simulink model "EurlerDynJointVerifyIdn"  (Simulink 7.6)
settings: Solver=ode45  StartTime=0.0  StopTime=8  RelTol=1e-3
InitFcn:
  | eval('Config')
values from neighbouring files (symbols this model uses):
  a2 = 0    [Config.m]    (also in CtrPlatformCfg.m)
  a3 = 0    [Config.m]    (also in CtrPlatformCfg.m)
  a4 = 0    [Config.m]    (also in CtrPlatformCfg.m)
  a5 = 90    [Config.m]    (also in CtrPlatformCfg.m)
  a6 = 0    [Config.m]    (also in CtrPlatformCfg.m)
  DH_EU = [266     300     0       0       1016     0      174 ... (first row only)    [DynEulerTest.m]
  freq = tvel/radius    (= 1)    [Config.m]    (also in CtrPlatformCfg.m)
  Ft_EU = [0;0;0;0;0;0]    [DynEulerTest.m]
  init_Endx = gd_init(1,4)    [Config.m]    (also in CtrPlatformCfg.m)
  init_Endy = gd_init(2,4)    [Config.m]    (also in CtrPlatformCfg.m)
  init_Endz = gd_init(3,4)    [Config.m]    (also in CtrPlatformCfg.m)
  init_Rot = gd_init(1:3,1:3)    [Config.m]    (also in CtrPlatformCfg.m)
  L = [l1 l2 l3 l4 l5 l6 l7 l8 l9]    [Config.m]    (also in CtrPlatformCfg.m)
  tvel = 120    [Config.m]    (also in CtrPlatformCfg.m)
undefined symbols (not defined in the file or in its folder): a1, DH_Min, Ft_Min, Param_EU, Param_Min
libraries: mblibv1 x35, simulink x9
(part 1 of 2)
settings Model: Creator=DAI Dan  LastModifiedBy=DAI Dan
settings SimMechanicsCC: VisOnUpdateDiagram=on  VisDuringSimulation=on

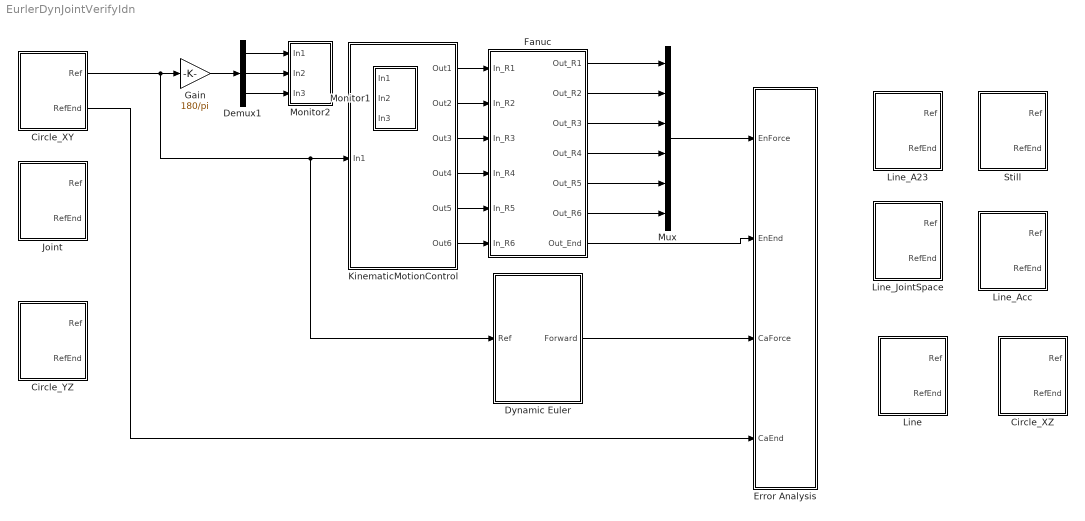
== system EurlerDynJointVerifyIdn ==
  Circle_XY : Subsystem
  Circle_XZ : Subsystem
  Circle_YZ : Subsystem
  Demux1 : Demux  Outputs=3
  Dynamic Euler : Subsystem
  Error Analysis : Subsystem
  Fanuc : Subsystem
  Gain : Gain  Gain=180/pi
  Joint : Subsystem
  KinematicMotionControl : Subsystem
  Line : Subsystem
  Line_A23 : Subsystem
  Line_Acc : Subsystem
  Line_JointSpace : Subsystem
  Monitor1 : Subsystem
  Monitor2 : Subsystem
  Mux : Mux  Inputs=6
  Still : Subsystem
  wires:
  KinematicMotionControl/1(Out1) -> Fanuc/1(In_R1)
  KinematicMotionControl/2(Out2) -> Fanuc/2(In_R2)
  KinematicMotionControl/3(Out3) -> Fanuc/3(In_R3)
  KinematicMotionControl/4(Out4) -> Fanuc/4(In_R4)
  KinematicMotionControl/5(Out5) -> Fanuc/5(In_R5)
  KinematicMotionControl/6(Out6) -> Fanuc/6(In_R6)
  Fanuc/5(Out_R5) -> Mux/5
  Fanuc/6(Out_R6) -> Mux/6
  Mux/1 -> Error Analysis/1(EnForce)
  Fanuc/4(Out_R4) -> Mux/4
  Fanuc/3(Out_R3) -> Mux/3
  Fanuc/2(Out_R2) -> Mux/2
  Fanuc/1(Out_R1) -> Mux/1
  Fanuc/7(Out_End) -> Error Analysis/2(EnEnd)
  Dynamic Euler/1(Forward) -> Error Analysis/3(CaForce)
  Demux1/1 -> Monitor2/1(In1)
  Demux1/2 -> Monitor2/2(In2)
  Demux1/3 -> Monitor2/3(In3)
  Gain/1 -> Demux1/1
  Circle_XY/1(Ref) -> Gain/1, KinematicMotionControl/1(In1), Dynamic Euler/1(Ref)
  Circle_XY/2(RefEnd) -> Error Analysis/4(CaEnd)

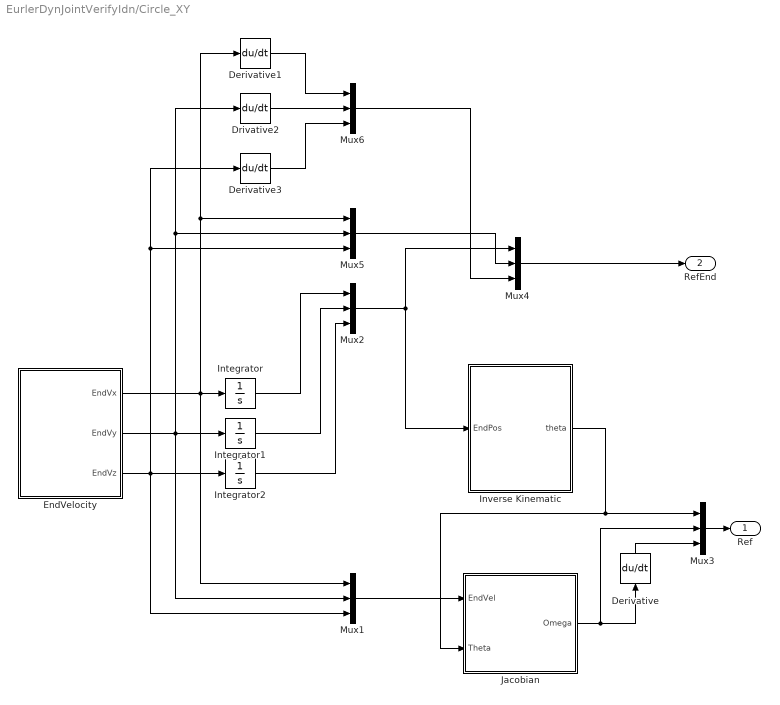
== system EurlerDynJointVerifyIdn/Circle_XY ==
  Derivative : Derivative
  Derivative1 : Derivative
  Derivative3 : Derivative
  Drivative2 : Derivative
  EndVelocity : Subsystem
  Integrator : Integrator  InitialCondition=init_Endx
  Integrator1 : Integrator  InitialCondition=init_Endy
  Integrator2 : Integrator  InitialCondition=init_Endz
  Inverse Kinematic : Stateflow chart  TreatAsAtomicUnit=on
  Jacobian : Stateflow chart  TreatAsAtomicUnit=on
  Mux{1..6} (6 alike) : Mux  Inputs=3
  Ref : Outport
  RefEnd : Outport  Port=2
  wires:
  Integrator/1 -> Mux2/1
  Integrator1/1 -> Mux2/2
  EndVelocity/1(EndVx) -> Integrator/1, Mux1/1, Mux5/1, Derivative1/1
  EndVelocity/2(EndVy) -> Integrator1/1, Mux1/2, Mux5/2, Drivative2/1
  EndVelocity/3(EndVz) -> Integrator2/1, Mux1/3, Mux5/3, Derivative3/1
  Integrator2/1 -> Mux2/3
  Mux2/1 -> Mux4/1, Inverse Kinematic/1(EndPos)
  Mux1/1 -> Jacobian/1(EndVel)
  Jacobian/1(Omega) -> Mux3/2, Derivative/1
  Mux3/1 -> Ref/1
  Derivative/1 -> Mux3/3
  Inverse Kinematic/1(theta) -> Mux3/1, Jacobian/2(Theta)
  Mux5/1 -> Mux4/2
  Mux4/1 -> RefEnd/1
  Derivative1/1 -> Mux6/1
  Drivative2/1 -> Mux6/2
  Derivative3/1 -> Mux6/3
  Mux6/1 -> Mux4/3

== system EurlerDynJointVerifyIdn/Circle_XZ ==
  Derivative : Derivative
  Derivative1 : Derivative
  Derivative3 : Derivative
  Drivative2 : Derivative
  EndVelocity : Subsystem
  Integrator : Integrator  InitialCondition=init_Endx
  Integrator1 : Integrator  InitialCondition=init_Endy
  Integrator2 : Integrator  InitialCondition=init_Endz
  Inverse Kinematic : Stateflow chart  TreatAsAtomicUnit=on
  Jacobian : Stateflow chart  TreatAsAtomicUnit=on
  Mux{1..6} (6 alike) : Mux  Inputs=3
  Ref : Outport
  RefEnd : Outport  Port=2
  wires:
  Integrator/1 -> Mux2/1
  Integrator1/1 -> Mux2/2
  EndVelocity/1(EndVx) -> Integrator/1, Mux1/1, Mux5/1, Derivative1/1
  EndVelocity/2(EndVy) -> Integrator1/1, Mux1/2, Mux5/2, Drivative2/1
  EndVelocity/3(EndVz) -> Integrator2/1, Mux1/3, Mux5/3, Derivative3/1
  Integrator2/1 -> Mux2/3
  Mux2/1 -> Mux4/1, Inverse Kinematic/1(EndPos)
  Mux1/1 -> Jacobian/1(EndVel)
  Jacobian/1(Omega) -> Mux3/2, Derivative/1
  Mux3/1 -> Ref/1
  Derivative/1 -> Mux3/3
  Inverse Kinematic/1(theta) -> Mux3/1, Jacobian/2(Theta)
  Mux5/1 -> Mux4/2
  Mux4/1 -> RefEnd/1
  Derivative1/1 -> Mux6/1
  Drivative2/1 -> Mux6/2
  Derivative3/1 -> Mux6/3
  Mux6/1 -> Mux4/3

== system EurlerDynJointVerifyIdn/Circle_YZ ==
  Derivative : Derivative
  Derivative1 : Derivative
  Derivative3 : Derivative
  Drivative2 : Derivative
  EndVelocity : Subsystem
  Integrator : Integrator  InitialCondition=init_Endx
  Integrator1 : Integrator  InitialCondition=init_Endy
  Integrator2 : Integrator  InitialCondition=init_Endz
  Inverse Kinematic : Stateflow chart  TreatAsAtomicUnit=on
  Jacobian : Stateflow chart  TreatAsAtomicUnit=on
  Mux{1..6} (6 alike) : Mux  Inputs=3
  Ref : Outport
  RefEnd : Outport  Port=2
  wires:
  Integrator/1 -> Mux2/1
  Integrator1/1 -> Mux2/2
  EndVelocity/1(EndVx) -> Integrator/1, Mux1/1, Mux5/1, Derivative1/1
  EndVelocity/2(EndVy) -> Integrator1/1, Mux1/2, Mux5/2, Drivative2/1
  EndVelocity/3(EndVz) -> Integrator2/1, Mux1/3, Mux5/3, Derivative3/1
  Integrator2/1 -> Mux2/3
  Mux2/1 -> Mux4/1, Inverse Kinematic/1(EndPos)
  Mux1/1 -> Jacobian/1(EndVel)
  Jacobian/1(Omega) -> Mux3/2, Derivative/1
  Mux3/1 -> Ref/1
  Derivative/1 -> Mux3/3
  Inverse Kinematic/1(theta) -> Mux3/1, Jacobian/2(Theta)
  Mux5/1 -> Mux4/2
  Mux4/1 -> RefEnd/1
  Derivative1/1 -> Mux6/1
  Drivative2/1 -> Mux6/2
  Derivative3/1 -> Mux6/3
  Mux6/1 -> Mux4/3

== system EurlerDynJointVerifyIdn/Dynamic Euler ==
  Ref : Inport
  Demux : Demux  Outputs=3
  Newton Euler Recursion : Stateflow chart  TreatAsAtomicUnit=on
  Newton Euler Recursion1 : Stateflow chart  TreatAsAtomicUnit=on
  To Workspace : ToWorkspace  VariableName=OutAngle1  SaveFormat=Structure With Time
  To Workspace1 : ToWorkspace  VariableName=OutOmega1  SaveFormat=Structure With Time
  To Workspace2 : ToWorkspace  VariableName=OutAcc1  SampleTime=-1  SaveFormat=Structure With Time
  Forward : Outport
  wires:
  Ref/1 -> Demux/1
  Demux/1 -> To Workspace/1, Newton Euler Recursion/1(Pos), Newton Euler Recursion1/1(Pos)
  Demux/2 -> To Workspace1/1, Newton Euler Recursion/2(Vel), Newton Euler Recursion1/2(Vel)
  Demux/3 -> To Workspace2/1, Newton Euler Recursion/3(Acc), Newton Euler Recursion1/3(Acc)
  Newton Euler Recursion1/1(Torque) -> Forward/1

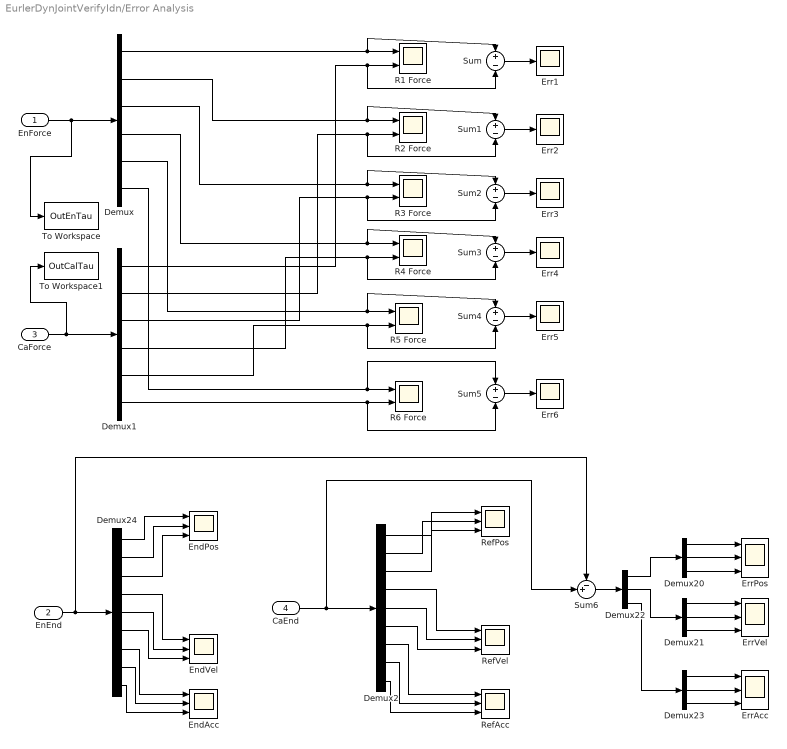
== system EurlerDynJointVerifyIdn/Error Analysis ==
  EnForce : Inport
  EnEnd : Inport  Port=2
  CaForce : Inport  Port=3
  CaEnd : Inport  Port=4
  Demux : Demux  Outputs=6
  Demux1 : Demux  Outputs=6
  Demux2 : Demux  Outputs=9
  Demux{20..23} (4 alike) : Demux  Outputs=3
  Demux24 : Demux  Outputs=9
  EndAcc : Scope  NumInputPorts=3
      settings: TimeRange=0.7279693486590038  YMin=-80~-80~0.03111111111111042  YMax=60~80~0.06666666666666621  SaveName=ScopeData12
  EndPos : Scope  NumInputPorts=3
      settings: TimeRange=10  YMin=1150~-100~1518.9999998  YMax=1350~200~1519.0000003  SaveName=ScopeData13
  EndVel : Scope  NumInputPorts=3
      settings: YMin=-5~-5~-5  YMax=5~5~5  SaveName=ScopeData14
  Err{1..6} (6 alike) : Scope
      Err1 settings: SaveName=ScopeData6
      Err2 settings: SaveName=ScopeData7
      Err3 settings: TimeRange=10  SaveName=ScopeData8
      Err4 settings: TimeRange=3  SaveName=ScopeData9
      Err5 settings: SaveName=ScopeData10
      Err6 settings: SaveName=ScopeData11
  ErrAcc : Scope  NumInputPorts=3
      settings: YMin=-5~-5~-5  YMax=5~5~5  SaveName=ScopeData15
  ErrPos : Scope  NumInputPorts=3
      settings: YMin=-5~-5~-5  YMax=5~5~5  SaveName=ScopeData16
  ErrVel : Scope  NumInputPorts=3
      settings: YMin=-5~-5~-5  YMax=5~5~5  SaveName=ScopeData17
  R1 Force : Scope  NumInputPorts=2
      settings: TimeRange=10  YMin=-2.999999999999999e-017~-1  YMax=4e-017~1
  R2 Force : Scope  NumInputPorts=2
      settings: YMin=-5~-5  YMax=5~5
  R3 Force : Scope  NumInputPorts=2
      settings: YMin=-5~-5  YMax=5~5  SaveName=ScopeData2
  R4 Force : Scope  NumInputPorts=2
      settings: TimeRange=8  YMin=-5~-5  YMax=5~5  SaveName=ScopeData3
  R5 Force : Scope  NumInputPorts=2
      settings: TimeRange=10  YMin=-4.18~4.060000000000001  YMax=-4.04~4.2  SaveName=ScopeData4
  R6 Force : Scope  NumInputPorts=2
      settings: TimeRange=10  YMin=-1.6e-006~-0.003  YMax=4e-007~0.004  SaveName=ScopeData5
  RefAcc : Scope  NumInputPorts=3
      settings: TimeRange=10  YMin=-5~-5~-5  YMax=5~5~5  SaveName=ScopeData18
  RefPos : Scope  NumInputPorts=3
      settings: YMin=-5~-5~-5  YMax=5~5~5  SaveName=ScopeData19
  RefVel : Scope  NumInputPorts=3
      settings: TimeRange=10  YMin=0~-1~-1  YMax=60~1~1  SaveName=ScopeData20
  Sum{,1..5} (6 alike) : Sum  Inputs=+|-
  Sum6 : Sum  Inputs=-+|
  To Workspace : ToWorkspace  VariableName=OutEnTau  SampleTime=-1  SaveFormat=Structure
  To Workspace1 : ToWorkspace  VariableName=OutCalTau  SampleTime=-1  SaveFormat=Structure
  wires:
  Sum/1 -> Err1/1
  Sum1/1 -> Err2/1
  Sum2/1 -> Err3/1
  Sum3/1 -> Err4/1
  Sum4/1 -> Err5/1
  Sum5/1 -> Err6/1
  EnForce/1 -> Demux/1, To Workspace/1
  CaForce/1 -> Demux1/1, To Workspace1/1
  Demux/1 -> Sum/1, R1 Force/1
  Demux1/1 -> Sum/2, R1 Force/2
  Demux/2 -> R2 Force/1, Sum1/1
  Demux/3 -> R3 Force/1, Sum2/1
  Demux/4 -> R4 Force/1, Sum3/1
  Demux/5 -> R5 Force/1, Sum4/1
  Demux/6 -> Sum5/1, R6 Force/1
  Demux1/2 -> R2 Force/2, Sum1/2
  Demux1/3 -> R3 Force/2, Sum2/2
  Demux1/4 -> R4 Force/2, Sum3/2
  Demux1/5 -> R5 Force/2, Sum4/2
  Demux1/6 -> Sum5/2, R6 Force/2
  EnEnd/1 -> Sum6/1, Demux24/1
  CaEnd/1 -> Sum6/2, Demux2/1
  Demux20/1 -> ErrPos/1
  Demux20/2 -> ErrPos/2
  Demux20/3 -> ErrPos/3
  Sum6/1 -> Demux22/1
  Demux22/1 -> Demux20/1
  Demux22/2 -> Demux21/1
  Demux21/1 -> ErrVel/1
  Demux21/2 -> ErrVel/2
  Demux21/3 -> ErrVel/3
  Demux2/1 -> RefPos/1
  Demux2/2 -> RefPos/2
  Demux2/3 -> RefPos/3
  Demux2/4 -> RefVel/1
  Demux2/5 -> RefVel/2
  Demux2/6 -> RefVel/3
  Demux2/7 -> RefAcc/1
  Demux2/8 -> RefAcc/2
  Demux2/9 -> RefAcc/3
  Demux23/1 -> ErrAcc/1
  Demux23/2 -> ErrAcc/2
  Demux23/3 -> ErrAcc/3
  Demux22/3 -> Demux23/1
  Demux24/1 -> EndPos/1
  Demux24/2 -> EndPos/2
  Demux24/3 -> EndPos/3
  Demux24/4 -> EndVel/1
  Demux24/5 -> EndVel/2
  Demux24/6 -> EndVel/3
  Demux24/7 -> EndAcc/1
  Demux24/8 -> EndAcc/2
  Demux24/9 -> EndAcc/3

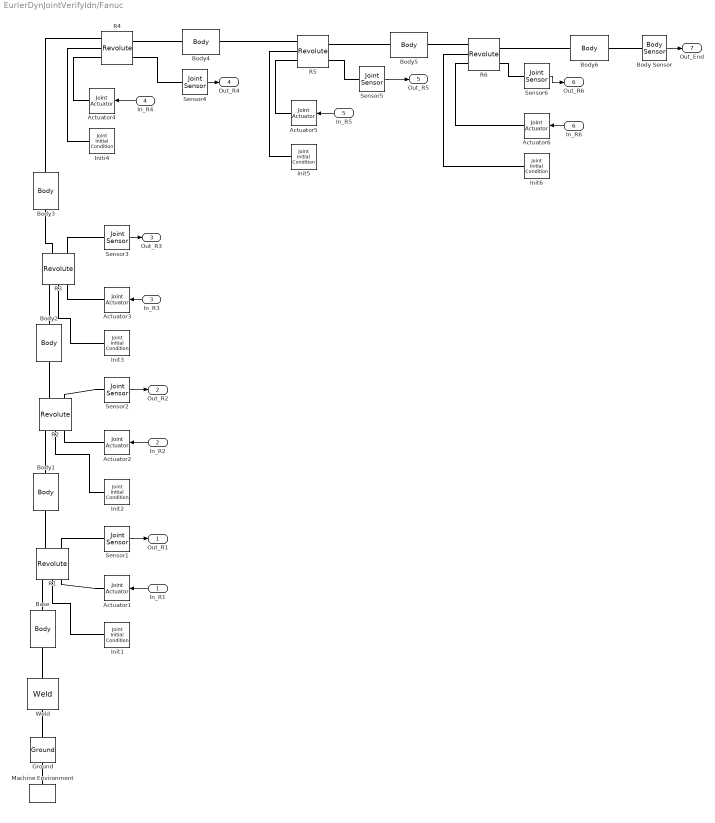
== system EurlerDynJointVerifyIdn/Fanuc ==
  In_R1 : Inport
  In_R2 : Inport  Port=2
  In_R3 : Inport  Port=3
  In_R4 : Inport  Port=4
  In_R5 : Inport  Port=5
  In_R6 : Inport  Port=6
  Actuator{1..6} (6 alike) : mblibv1/Sensors &  Actuators/Joint Actuator  DialogController=MECH.DynMechDlgSource  SystemSampleTime=-1  UpdateFromCAD=off  PhysicalDomain=Mechanical  PortType=blob  ActuationStyle=Motion  AngleUnits=rad  ArcVelocityUnits=rad/s  ArcAccelerationUnits=rad/s^2  CoordPositionUnits=m  VelocityUnits=m/s  AccelerationUnits=m/s^2  ForceUnits=N  TorqueUnits=N*m  ActiveIO=on  Width=3  DialogClass=MechanicalActuatorBlock  Primitive=R1  ReferenceFrame=Absolute (World)
  Base : mblibv1/Bodies/Body  DialogController=MECH.DynMechDlgSource  PhysicalDomain=mechanical  SubClassName=Unknown  LeftPortType=workingframe  RightPortType=workingframe  LConnTagsString=CS1  RConnTagsString=CS2  UpdateFromCAD=on  DialogClass=MechanicalBodyBlock  Mass=133.95  MassUnits=kg  InertiaUnits=kg*m^2  Inertia=[3.0977 0.0155 -0.0939;0.0155 3.3580 0.0061;-0.0939 0.0061 5.1969]  Shape=Cylinder  ShapeDims=[1 1]  ShapeUnits=m  ShapeUse=false  Density=1  DensityUnits=kg/m^3  DensityUse=false  GraphicsMode=GFXFILE  GraphicsFileName=M-710iC50 M-710iC70 - M-710iC50 M-710iC70 base-1.STL  BodyColorSelMode=COLORPALETTE  BodyColor=[0.25098 0.25098 0.25098]  AttachedToCS=CS1  CG=Right$CG$[-0.0437 -0.0026 0.1059]$WORLD$WORLD$m$[1 0 0;0 1 0;0 0 1]$3x3 Transform$rad$WORLD$false$none  WorkingFrames=Left$CS1$[0 0 0]$WORLD$WORLD$m$[1 0 0;0 1 0;0 0 1]$3x3 Transform$rad$WORLD$true$none#Right$CS2$[0 0 0.266]$WORLD$WORLD$m$[1 0 0;0 1 0;0 0 1]$3x3 Transform$rad$WORLD$true$none  CGPos=[-0.0437 -0.0026 0.1059]  CGRot=[1 0 0;0 1 0;0 0 1]  CS0Pos=[]  CS0Rot=[]  CS1Pos=[0 0 0]  CS1Rot=[1 0 0;0 1 0;0 0 1]  CS2Pos=[0 0 0.266]  CS2Rot=[1 0 0;0 1 0;0 0 1]  CS3Pos=[]  CS3Rot=[]  CS4Pos=[]  CS4Rot=[]  CS5Pos=[]  CS5Rot=[]  CS6Pos=[]  CS6Rot=[]  CS7Pos=[]  CS7Rot=[]  CS8Pos=[]  CS8Rot=[]  CS9Pos=[]  CS9Rot=[]  CS10Pos=[]  CS10Rot=[]  CS11Pos=[]  CS11Rot=[]  CS12Pos=[]  CS12Rot=[]  CS13Pos=[]  CS13Rot=[]  CS14Pos=[]  CS14Rot=[]  CS15Pos=[]  CS15Rot=[]  CS16Pos=[]  CS16Rot=[]  CS17Pos=[]  CS17Rot=[]  CS18Pos=[]  CS18Rot=[]  CS19Pos=[]  CS19Rot=[]  CS20Pos=[]  CS20Rot=[]
  Body Sensor : mblibv1/Sensors &  Actuators/Body Sensor  DialogController=MECH.DynMechDlgSource  SystemSampleTime=-1  UpdateFromCAD=off  PhysicalDomain=Mechanical  PortType=blob  Muxed=on  Pose=off  Angle=on  AngleUnits=deg  ArcVelocity=off  ArcVelocityUnits=deg/s  ArcAcceleration=off  ArcAccelerationUnits=deg/s^2  CoordPosition=on  CoordPositionUnits=mm  Velocity=on  VelocityUnits=mm/s  Acceleration=on  AccelerationUnits=mm/s^2  Quaternion=on  QuaternionDT=off  QuaternionDDT=off  QuaternionUnits=off  OutputVector=[1]  ActiveIO=on  Width=9  DialogClass=MechanicalSensorBlock  ReferenceFrame=Absolute (World)
  Body1 : mblibv1/Bodies/Body  DialogController=MECH.DynMechDlgSource  PhysicalDomain=mechanical  SubClassName=Unknown  LeftPortType=workingframe  RightPortType=workingframe  LConnTagsString=CS2  RConnTagsString=CS3  UpdateFromCAD=on  DialogClass=MechanicalBodyBlock  Mass=170.31  MassUnits=kg  InertiaUnits=kg*m^2  Inertia=[5.2954 -0.2565 -0.6366;-0.2565 4.7000 0.2830;-0.6366 0.2829 5.8635]  Shape=Cylinder  ShapeDims=[1 1]  ShapeUnits=m  ShapeUse=false  Density=1  DensityUnits=kg/m^3  DensityUse=false  GraphicsMode=GFXFILE  GraphicsFileName=M-710iC50 M-710iC70 - M-710iC50 M-710iC70 axis1-1.STL  BodyColorSelMode=COLORPALETTE  BodyColor=[0.86667 0.86667 0.8902]  AttachedToCS=CS1  CG=Right$CG$[0.0407 -0.0528 0.4702]$WORLD$WORLD$m$[1 0 0;0 1 0;0 0 1]$3x3 Transform$rad$WORLD$false$none  WorkingFrames=Right$CS1$[0 0 0]$WORLD$WORLD$m$[1 0 0;0 1 0;0 0 1]$3x3 Transform$rad$WORLD$false$none#Left$CS2$[0 0 0.266]$WORLD$WORLD$m$[1 0 0;0 1 0;0 0 1]$3x3 Transform$rad$WORLD$true$none#Right$CS3$[0.15 0.062 0.566]$WORLD$WORLD$m$[1 0 0;0 1 0;0 0 1]$3x3 Transform$rad$WORLD$true$none  CGPos=[0.0407 -0.0528 0.4702]  CGRot=[1 0 0;0 1 0;0 0 1]  CS0Pos=[]  CS0Rot=[]  CS1Pos=[0 0 0]  CS1Rot=[1 0 0;0 1 0;0 0 1]  CS2Pos=[0 0 0.266]  CS2Rot=[1 0 0;0 1 0;0 0 1]  CS3Pos=[0.15 0.062 0.566]  CS3Rot=[1 0 0;0 1 0;0 0 1]  CS4Pos=[]  CS4Rot=[]  CS5Pos=[]  CS5Rot=[]  CS6Pos=[]  CS6Rot=[]  CS7Pos=[]  CS7Rot=[]  CS8Pos=[]  CS8Rot=[]  CS9Pos=[]  CS9Rot=[]  CS10Pos=[]  CS10Rot=[]  CS11Pos=[]  CS11Rot=[]  CS12Pos=[]  CS12Rot=[]  CS13Pos=[]  CS13Rot=[]  CS14Pos=[]  CS14Rot=[]  CS15Pos=[]  CS15Rot=[]  CS16Pos=[]  CS16Rot=[]  CS17Pos=[]  CS17Rot=[]  CS18Pos=[]  CS18Rot=[]  CS19Pos=[]  CS19Rot=[]  CS20Pos=[]  CS20Rot=[]
  Body2 : mblibv1/Bodies/Body  DialogController=MECH.DynMechDlgSource  PhysicalDomain=mechanical  SubClassName=Unknown  LeftPortType=workingframe  RightPortType=workingframe  LConnTagsString=CS2  RConnTagsString=CS3  UpdateFromCAD=on  DialogClass=MechanicalBodyBlock  Mass=63.74  MassUnits=kg  InertiaUnits=kg*m^2  Inertia=[5.8840 0.0072 0.0135;0.0072 6.0178 -0.1907;0.0135 -0.1907 0.3374]  Shape=Cylinder  ShapeDims=[1 1]  ShapeUnits=m  ShapeUse=false  Density=1  DensityUnits=kg/m^3  DensityUse=false  GraphicsMode=GFXFILE  GraphicsFileName=M-710iC50 M-710iC70 - M-710iC50 M-710iC70 axis2-1.STL  BodyColorSelMode=COLORPALETTE  BodyColor=[1 1 0]  AttachedToCS=CS1  CG=Right$CG$[0.1510 0.1746 0.9687]$WORLD$WORLD$m$[1 0 0;0 1 0;0 0 1]$3x3 Transform$rad$WORLD$false$none  WorkingFrames=Right$CS1$[0 0 0]$WORLD$WORLD$m$[1 0 0;0 1 0;0 0 1]$3x3 Transform$rad$WORLD$false$none#Left$CS2$[0.15 0.062 0.566]$WORLD$WORLD$m$[1 0 0;0 1 0;0 0 1]$3x3 Transform$rad$WORLD$true$none#Right$CS3$[0.15 0.227 1.436]$WORLD$WORLD$m$[1 0 0;0 1 0;0 0 1]$3x3 Transform$rad$WORLD$true$none  CGPos=[0.1510 0.1746 0.9687]  CGRot=[1 0 0;0 1 0;0 0 1]  CS0Pos=[]  CS0Rot=[]  CS1Pos=[0 0 0]  CS1Rot=[1 0 0;0 1 0;0 0 1]  CS2Pos=[0.15 0.062 0.566]  CS2Rot=[1 0 0;0 1 0;0 0 1]  CS3Pos=[0.15 0.227 1.436]  CS3Rot=[1 0 0;0 1 0;0 0 1]  CS4Pos=[]  CS4Rot=[]  CS5Pos=[]  CS5Rot=[]  CS6Pos=[]  CS6Rot=[]  CS7Pos=[]  CS7Rot=[]  CS8Pos=[]  CS8Rot=[]  CS9Pos=[]  CS9Rot=[]  CS10Pos=[]  CS10Rot=[]  CS11Pos=[]  CS11Rot=[]  CS12Pos=[]  CS12Rot=[]  CS13Pos=[]  CS13Rot=[]  CS14Pos=[]  CS14Rot=[]  CS15Pos=[]  CS15Rot=[]  CS16Pos=[]  CS16Rot=[]  CS17Pos=[]  CS17Rot=[]  CS18Pos=[]  CS18Rot=[]  CS19Pos=[]  CS19Rot=[]  CS20Pos=[]  CS20Rot=[]
  Body3 : mblibv1/Bodies/Body  DialogController=MECH.DynMechDlgSource  PhysicalDomain=mechanical  SubClassName=Unknown  LeftPortType=workingframe  RightPortType=workingframe  LConnTagsString=CS2  RConnTagsString=CS3  UpdateFromCAD=on  DialogClass=MechanicalBodyBlock  Mass=98.98  MassUnits=kg  InertiaUnits=kg*m^2  Inertia=[1.8201 -0.2274 -0.3112;-0.2274 2.2537 -0.1441;-0.3112 -0.1441 1.9485]  Shape=Cylinder  ShapeDims=[1 1]  ShapeUnits=m  ShapeUse=false  Density=1  DensityUnits=kg/m^3  DensityUse=false  GraphicsMode=GFXFILE  GraphicsFileName=M-710iC50 M-710iC70 - M-710iC50 M-710iC70 axis3-1.STL  BodyColorSelMode=COLORPALETTE  BodyColor=[1 1 0]  AttachedToCS=CS1  CG=Right$CG$[0.1568 -0.0318 1.5191]$WORLD$WORLD$m$[1 0 0;0 1 0;0 0 1]$3x3 Transform$rad$WORLD$false$none  WorkingFrames=Right$CS1$[0 0 0]$WORLD$WORLD$m$[1 0 0;0 1 0;0 0 1]$3x3 Transform$rad$WORLD$false$none#Left$CS2$[0.15 0.227 1.436]$WORLD$WORLD$m$[1 0 0;0 1 0;0 0 1]$3x3 Transform$rad$WORLD$true$none#Right$CS3$[0.4525 0 1.606]$WORLD$WORLD$m$[1 0 0;0 1 0;0 0 1]$3x3 Transform$rad$WORLD$true$none  CGPos=[0.1568 -0.0318 1.5191]  CGRot=[1 0 0;0 1 0;0 0 1]  CS0Pos=[]  CS0Rot=[]  CS1Pos=[0 0 0]  CS1Rot=[1 0 0;0 1 0;0 0 1]  CS2Pos=[0.15 0.227 1.436]  CS2Rot=[1 0 0;0 1 0;0 0 1]  CS3Pos=[0.4525 0 1.606]  CS3Rot=[1 0 0;0 1 0;0 0 1]  CS4Pos=[]  CS4Rot=[]  CS5Pos=[]  CS5Rot=[]  CS6Pos=[]  CS6Rot=[]  CS7Pos=[]  CS7Rot=[]  CS8Pos=[]  CS8Rot=[]  CS9Pos=[]  CS9Rot=[]  CS10Pos=[]  CS10Rot=[]  CS11Pos=[]  CS11Rot=[]  CS12Pos=[]  CS12Rot=[]  CS13Pos=[]  CS13Rot=[]  CS14Pos=[]  CS14Rot=[]  CS15Pos=[]  CS15Rot=[]  CS16Pos=[]  CS16Rot=[]  CS17Pos=[]  CS17Rot=[]  CS18Pos=[]  CS18Rot=[]  CS19Pos=[]  CS19Rot=[]  CS20Pos=[]  CS20Rot=[]
  Body4 : mblibv1/Bodies/Body  DialogController=MECH.DynMechDlgSource  PhysicalDomain=mechanical  SubClassName=Unknown  LeftPortType=workingframe  RightPortType=workingframe  LConnTagsString=CS2  RConnTagsString=CS3  UpdateFromCAD=on  DialogClass=MechanicalBodyBlock  Mass=24.46  MassUnits=kg  InertiaUnits=kg*m^2  Inertia=[0.0607 -0.0922 0;-0.0922 1.4493 0;0 0,1.4620]  Shape=Cylinder  ShapeDims=[1 1]  ShapeUnits=m  ShapeUse=false  Density=1  DensityUnits=kg/m^3  DensityUse=false  GraphicsMode=GFXFILE  GraphicsFileName=M-710iC50 M-710iC70 - M-710iC50 M-710iC70 axis4-1.STL  BodyColorSelMode=COLORPALETTE  BodyColor=[1 1 0]  AttachedToCS=CS1  CG=Right$CG$[0.8245 -0.0110 1.606]$WORLD$WORLD$m$[1 0 0;0 1 0;0 0 1]$3x3 Transform$rad$WORLD$false$none  WorkingFrames=Right$CS1$[0.4525 0 1.606]$WORLD$WORLD$m$[1 0 0;0 0 1;0 -1 0]$3x3 Transform$rad$WORLD$false$none#Left$CS2$[0.4525 0 1.606]$WORLD$WORLD$m$[1 0 0;0 1 0;0 0 1]$3x3 Transform$rad$WORLD$true$none#Right$CS3$[1.166 -0.113 1.606]$WORLD$WORLD$m$[1 0 0;0 1 0;0 0 1]$3x3 Transform$rad$WORLD$true$none  CGPos=[0.8245 -0.0110 1.606]  CGRot=[1 0 0;0 1 0;0 0 1]  CS0Pos=[]  CS0Rot=[]  CS1Pos=[0.4525 0 1.606]  CS1Rot=[1 0 0;0 0 1;0 -1 0]  CS2Pos=[0.4525 0 1.606]  CS2Rot=[1 0 0;0 1 0;0 0 1]  CS3Pos=[1.166 -0.113 1.606]  CS3Rot=[1 0 0;0 1 0;0 0 1]  CS4Pos=[]  CS4Rot=[]  CS5Pos=[]  CS5Rot=[]  CS6Pos=[]  CS6Rot=[]  CS7Pos=[]  CS7Rot=[]  CS8Pos=[]  CS8Rot=[]  CS9Pos=[]  CS9Rot=[]  CS10Pos=[]  CS10Rot=[]  CS11Pos=[]  CS11Rot=[]  CS12Pos=[]  CS12Rot=[]  CS13Pos=[]  CS13Rot=[]  CS14Pos=[]  CS14Rot=[]  CS15Pos=[]  CS15Rot=[]  CS16Pos=[]  CS16Rot=[]  CS17Pos=[]  CS17Rot=[]  CS18Pos=[]  CS18Rot=[]  CS19Pos=[]  CS19Rot=[]  CS20Pos=[]  CS20Rot=[]
  Body5 : mblibv1/Bodies/Body  DialogController=MECH.DynMechDlgSource  PhysicalDomain=mechanical  SubClassName=Unknown  LeftPortType=workingframe  RightPortType=workingframe  LConnTagsString=CS2  RConnTagsString=CS3  UpdateFromCAD=on  DialogClass=MechanicalBodyBlock  Mass=5.24  MassUnits=kg  InertiaUnits=kg*m^2  Inertia=[0.0191 0.0032 0;0.0032 0.0228 0;0 0 0.0291]  Shape=Cylinder  ShapeDims=[1 1]  ShapeUnits=m  ShapeUse=false  Density=1  DensityUnits=kg/m^3  DensityUse=false  GraphicsMode=GFXFILE  GraphicsFileName=M-710iC50 M-710iC70 - M-710iC50 M-710iC70 axis5-1.STL  BodyColorSelMode=COLORPALETTE  BodyColor=[1 1 0]  AttachedToCS=CS1  CG=Right$CG$[1.2407 0.0180 1.606]$WORLD$WORLD$m$[1 0 0;0 1 0;0 0 1]$3x3 Transform$rad$WORLD$false$none  WorkingFrames=Right$CS1$[0 0 0]$WORLD$WORLD$m$[1 0 0;0 1 0;0 0 1]$3x3 Transform$rad$WORLD$false$none#Left$CS2$[1.166 -0.113 1.606]$WORLD$WORLD$m$[1 0 0;0 1 0;0 0 1]$3x3 Transform$rad$WORLD$true$none#Right$CS3$[1.320 0 1.606]$WORLD$WORLD$m$[1 0 0;0 1 0;0 0 1]$3x3 Transform$rad$WORLD$true$none  CGPos=[1.2407 0.0180 1.606]  CGRot=[1 0 0;0 1 0;0 0 1]  CS0Pos=[]  CS0Rot=[]  CS1Pos=[0 0 0]  CS1Rot=[1 0 0;0 1 0;0 0 1]  CS2Pos=[1.166 -0.113 1.606]  CS2Rot=[1 0 0;0 1 0;0 0 1]  CS3Pos=[1.320 0 1.606]  CS3Rot=[1 0 0;0 1 0;0 0 1]  CS4Pos=[]  CS4Rot=[]  CS5Pos=[]  CS5Rot=[]  CS6Pos=[]  CS6Rot=[]  CS7Pos=[]  CS7Rot=[]  CS8Pos=[]  CS8Rot=[]  CS9Pos=[]  CS9Rot=[]  CS10Pos=[]  CS10Rot=[]  CS11Pos=[]  CS11Rot=[]  CS12Pos=[]  CS12Rot=[]  CS13Pos=[]  CS13Rot=[]  CS14Pos=[]  CS14Rot=[]  CS15Pos=[]  CS15Rot=[]  CS16Pos=[]  CS16Rot=[]  CS17Pos=[]  CS17Rot=[]  CS18Pos=[]  CS18Rot=[]  CS19Pos=[]  CS19Rot=[]  CS20Pos=[]  CS20Rot=[]
  Body6 : mblibv1/Bodies/Body  DialogController=MECH.DynMechDlgSource  PhysicalDomain=mechanical  SubClassName=Unknown  LeftPortType=workingframe  RightPortType=workingframe  LConnTagsString=CS2  RConnTagsString=CS3  UpdateFromCAD=on  DialogClass=MechanicalBodyBlock  Mass=0.6  MassUnits=kg  InertiaUnits=kg*m^2  Inertia=[0.0012 0 0;0 0.0007 0;0 0 0.0007]  Shape=Cylinder  ShapeDims=[1 1]  ShapeUnits=m  ShapeUse=false  Density=1  DensityUnits=kg/m^3  DensityUse=false  GraphicsMode=GFXFILE  GraphicsFileName=M-710iC50 M-710iC70 - M-710iC50 M-710iC70 axis6-1.STL  BodyColorSelMode=COLORPALETTE  BodyColor=[0.75294 0.75294 0.75294]  AttachedToCS=CS1  CG=Right$CG$[1.330 0 1.606]$WORLD$WORLD$m$[1 0 0;0 1 0;0 0 1]$3x3 Transform$rad$WORLD$false$none  WorkingFrames=Right$CS1$[1.34 0 1.606]$WORLD$WORLD$m$[0 0 1;0 -1 0;1 0 0]$3x3 Transform$rad$WORLD$false$none#Left$CS2$[1.320 0 1.606]$WORLD$WORLD$m$[1 0 0;0 1 0;0 0 1]$3x3 Transform$rad$WORLD$true$none#Right$CS3$[1.34 0 1.606]$WORLD$WORLD$m$[1 0 0;0 1 0;0 0 1]$3x3 Transform$rad$WORLD$true$none  CGPos=[1.330 0 1.606]  CGRot=[1 0 0;0 1 0;0 0 1]  CS0Pos=[]  CS0Rot=[]  CS1Pos=[1.34 0 1.606]  CS1Rot=[0 0 1;0 -1 0;1 0 0]  CS2Pos=[1.320 0 1.606]  CS2Rot=[1 0 0;0 1 0;0 0 1]  CS3Pos=[1.34 0 1.606]  CS3Rot=[1 0 0;0 1 0;0 0 1]  CS4Pos=[]  CS4Rot=[]  CS5Pos=[]  CS5Rot=[]  CS6Pos=[]  CS6Rot=[]  CS7Pos=[]  CS7Rot=[]  CS8Pos=[]  CS8Rot=[]  CS9Pos=[]  CS9Rot=[]  CS10Pos=[]  CS10Rot=[]  CS11Pos=[]  CS11Rot=[]  CS12Pos=[]  CS12Rot=[]  CS13Pos=[]  CS13Rot=[]  CS14Pos=[]  CS14Rot=[]  CS15Pos=[]  CS15Rot=[]  CS16Pos=[]  CS16Rot=[]  CS17Pos=[]  CS17Rot=[]  CS18Pos=[]  CS18Rot=[]  CS19Pos=[]  CS19Rot=[]  CS20Pos=[]  CS20Rot=[]
  Ground : mblibv1/Bodies/Ground  DialogController=MECH.DynMechDlgSource  SystemSampleTime=-1  UpdateFromCAD=on  LeftPortType=env  RightPortType=workingframe  PhysicalDomain=Mechanical  DialogClass=GroundBlock  CoordPosition=[0 0 0]  CoordPositionUnits=m  StateVectorMgrId=1  MachineId=[2 0]  ShowEnvPort=on
  Init1 : mblibv1/Sensors &  Actuators/Joint Initial Condition  DialogController=MECH.DynMechDlgSource  SystemSampleTime=-1  UpdateFromCAD=off  LeftPortType=blob  RightPortType=blob  PhysicalDomain=mechanical  DialogClass=InitialConditionBlock  InitialConditions=P1$false$0$m$deg$0$m/s$deg/s#P2$false$0$m$deg$0$m/s$deg/s#P3$false$0$m$deg$0$m/s$deg/s#R1$true$a1$m$deg$0$m/s$deg/s#R2$false$0$m$deg$0$m/s$deg/s#R3$false$0$m$deg$0$m/s$deg/s#S$false$0$m$deg$0$m/s$deg/s  P1PIC=0  P1VIC=0  P2PIC=0  P2VIC=0  P3PIC=0  P3VIC=0  R1PIC=a1  R1VIC=0  R2PIC=0  R2VIC=0  R3PIC=0  R3VIC=0  SPIC=0  SVIC=0
  Init2 : mblibv1/Sensors &  Actuators/Joint Initial Condition  DialogController=MECH.DynMechDlgSource  SystemSampleTime=-1  UpdateFromCAD=off  LeftPortType=blob  RightPortType=blob  PhysicalDomain=mechanical  DialogClass=InitialConditionBlock  InitialConditions=P1$false$0$m$deg$0$m/s$deg/s#P2$false$0$m$deg$0$m/s$deg/s#P3$false$0$m$deg$0$m/s$deg/s#R1$true$a2$m$deg$0$m/s$deg/s#R2$false$0$m$deg$0$m/s$deg/s#R3$false$0$m$deg$0$m/s$deg/s#S$false$0$m$deg$0$m/s$deg/s  P1PIC=0  P1VIC=0  P2PIC=0  P2VIC=0  P3PIC=0  P3VIC=0  R1PIC=a2  R1VIC=0  R2PIC=0  R2VIC=0  R3PIC=0  R3VIC=0  SPIC=0  SVIC=0
  Init3 : mblibv1/Sensors &  Actuators/Joint Initial Condition  DialogController=MECH.DynMechDlgSource  SystemSampleTime=-1  UpdateFromCAD=off  LeftPortType=blob  RightPortType=blob  PhysicalDomain=mechanical  DialogClass=InitialConditionBlock  InitialConditions=P1$false$0$m$deg$0$m/s$deg/s#P2$false$0$m$deg$0$m/s$deg/s#P3$false$0$m$deg$0$m/s$deg/s#R1$true$a3$m$deg$0$m/s$deg/s#R2$false$0$m$deg$0$m/s$deg/s#R3$false$0$m$deg$0$m/s$deg/s#S$false$0$m$deg$0$m/s$deg/s  P1PIC=0  P1VIC=0  P2PIC=0  P2VIC=0  P3PIC=0  P3VIC=0  R1PIC=a3  R1VIC=0  R2PIC=0  R2VIC=0  R3PIC=0  R3VIC=0  SPIC=0  SVIC=0
  Init5 : mblibv1/Sensors &  Actuators/Joint Initial Condition  DialogController=MECH.DynMechDlgSource  SystemSampleTime=-1  UpdateFromCAD=off  LeftPortType=blob  RightPortType=blob  PhysicalDomain=mechanical  DialogClass=InitialConditionBlock  InitialConditions=P1$false$0$m$deg$0$m/s$deg/s#P2$false$0$m$deg$0$m/s$deg/s#P3$false$0$m$deg$0$m/s$deg/s#R1$true$a5$m$deg$0$m/s$deg/s#R2$false$0$m$deg$0$m/s$deg/s#R3$false$0$m$deg$0$m/s$deg/s#S$false$0$m$deg$0$m/s$deg/s  P1PIC=0  P1VIC=0  P2PIC=0  P2VIC=0  P3PIC=0  P3VIC=0  R1PIC=a5  R1VIC=0  R2PIC=0  R2VIC=0  R3PIC=0  R3VIC=0  SPIC=0  SVIC=0
  Init6 : mblibv1/Sensors &  Actuators/Joint Initial Condition  DialogController=MECH.DynMechDlgSource  SystemSampleTime=-1  UpdateFromCAD=off  LeftPortType=blob  RightPortType=blob  PhysicalDomain=mechanical  DialogClass=InitialConditionBlock  InitialConditions=P1$false$0$m$deg$0$m/s$deg/s#P2$false$0$m$deg$0$m/s$deg/s#P3$false$0$m$deg$0$m/s$deg/s#R1$true$a6$m$deg$0$m/s$deg/s#R2$false$0$m$deg$0$m/s$deg/s#R3$false$0$m$deg$0$m/s$deg/s#S$false$0$m$deg$0$m/s$deg/s  P1PIC=0  P1VIC=0  P2PIC=0  P2VIC=0  P3PIC=0  P3VIC=0  R1PIC=a6  R1VIC=0  R2PIC=0  R2VIC=0  R3PIC=0  R3VIC=0  SPIC=0  SVIC=0
  Initi4 : mblibv1/Sensors &  Actuators/Joint Initial Condition  DialogController=MECH.DynMechDlgSource  SystemSampleTime=-1  UpdateFromCAD=off  LeftPortType=blob  RightPortType=blob  PhysicalDomain=mechanical  DialogClass=InitialConditionBlock  InitialConditions=P1$false$0$m$deg$0$m/s$deg/s#P2$false$0$m$deg$0$m/s$deg/s#P3$false$0$m$deg$0$m/s$deg/s#R1$true$a4$m$deg$0$m/s$deg/s#R2$false$0$m$deg$0$m/s$deg/s#R3$false$0$m$deg$0$m/s$deg/s#S$false$0$m$deg$0$m/s$deg/s  P1PIC=0  P1VIC=0  P2PIC=0  P2VIC=0  P3PIC=0  P3VIC=0  R1PIC=a4  R1VIC=0  R2PIC=0  R2VIC=0  R3PIC=0  R3VIC=0  SPIC=0  SVIC=0
  Machine Environment : mblibv1/Bodies/Machine Environment  DialogController=MECH.DialogSource  SystemSampleTime=-1  PortType=env  PhysicalDomain=Mechanical  DialogTemplateClass=MECH.MachineEnvironment  SyncWhenCopied=off  Gravity=[0 0 -9.8]  GravityUnits=m/s^2  GravityAsSignal=off  Dimensionality=Auto-detect  AnalysisType=Inverse dynamics  LinearAssemblyTolerance=1e-3  LinearAssemblyToleranceUnits=m  AngularAssemblyTolerance=1e-3  AngularAssemblyToleranceUnits=rad  ConstraintSolverType=Stabilizing  ConstraintRelTolerance=1e-4  ConstraintAbsTolerance=1e-4  UseRobustSingularityHandling=off  RedundancyAnalysisToleranceType=Automatically select tolerance  RedundancyAnalysisTolerance=1e-14  StatePerturbationType=Fixed  PerturbationSize=1e-5  VisualizeMachine=on  BodyVisualizationType=Use model default body geometries  BodyColorSelMode=Use model default  DefaultBodyColor=[1 0 0]
  R1 : mblibv1/Joints/Revolute  DialogController=MECH.DynMechDlgSource  PhysicalDomain=mechanical  SubClassName=Unknown  LeftPortType=blob  RightPortType=blob  LConnTagsString=__newl0|SA1|SA2  RConnTagsString=__newr0|SA1  UpdateFromCAD=on  NumSAPorts=3  CutJoint=off  MarkAsCut=off  Primitives=prismatic  PrimitiveProps=R1$World$[0,0,1]$revolute  DialogClass=JointBlock  R1Axis=[0,0,1]
  R2 : mblibv1/Joints/Revolute  DialogController=MECH.DynMechDlgSource  PhysicalDomain=mechanical  SubClassName=Unknown  LeftPortType=blob  RightPortType=blob  LConnTagsString=__newl0|SA1|SA2  RConnTagsString=__newr0|SA1  UpdateFromCAD=on  NumSAPorts=3  CutJoint=off  MarkAsCut=off  Primitives=prismatic  PrimitiveProps=R1$World$[0,1,0]$revolute  DialogClass=JointBlock  R1Axis=[0,1,0]
  R3 : mblibv1/Joints/Revolute  DialogController=MECH.DynMechDlgSource  PhysicalDomain=mechanical  SubClassName=Unknown  LeftPortType=blob  RightPortType=blob  LConnTagsString=__newl0|SA1|SA2  RConnTagsString=__newr0|SA1  UpdateFromCAD=on  NumSAPorts=3  CutJoint=off  MarkAsCut=off  Primitives=prismatic  PrimitiveProps=R1$World$[0,1,0]$revolute  DialogClass=JointBlock  R1Axis=[0,1,0]
  R4 : mblibv1/Joints/Revolute  DialogController=MECH.DynMechDlgSource  PhysicalDomain=mechanical  SubClassName=Unknown  LeftPortType=blob  RightPortType=blob  LConnTagsString=__newl0|SA1|SA2  RConnTagsString=__newr0|SA1  UpdateFromCAD=on  NumSAPorts=3  CutJoint=off  MarkAsCut=off  Primitives=prismatic  PrimitiveProps=R1$World$[1,0,0]$revolute  DialogClass=JointBlock  R1Axis=[1,0,0]
  R5 : mblibv1/Joints/Revolute  DialogController=MECH.DynMechDlgSource  PhysicalDomain=mechanical  SubClassName=Unknown  LeftPortType=blob  RightPortType=blob  LConnTagsString=__newl0|SA1|SA2  RConnTagsString=__newr0|SA1  UpdateFromCAD=on  NumSAPorts=3  CutJoint=off  MarkAsCut=off  Primitives=prismatic  PrimitiveProps=R1$World$[0,1,0]$revolute  DialogClass=JointBlock  R1Axis=[0,1,0]
  R6 : mblibv1/Joints/Revolute  DialogController=MECH.DynMechDlgSource  PhysicalDomain=mechanical  SubClassName=Unknown  LeftPortType=blob  RightPortType=blob  LConnTagsString=__newl0|SA1|SA2  RConnTagsString=__newr0|SA1  UpdateFromCAD=on  NumSAPorts=3  CutJoint=off  MarkAsCut=off  Primitives=prismatic  PrimitiveProps=R1$World$[1,0,0]$revolute  DialogClass=JointBlock  R1Axis=[1,0,0]
  Sensor{1..6} (6 alike) : mblibv1/Sensors &  Actuators/Joint Sensor  DialogController=MECH.DynMechDlgSource  SystemSampleTime=-1  UpdateFromCAD=off  PhysicalDomain=Mechanical  PortType=blob  Muxed=on  Pose=off  Angle=off  AngleUnits=deg  ArcVelocity=off  ArcVelocityUnits=deg/s  ArcAcceleration=off  ArcAccelerationUnits=deg/s^2  CoordPosition=on  CoordPositionUnits=m  Velocity=off  VelocityUnits=m/s  Acceleration=off  AccelerationUnits=m/s^2  Quaternion=on  QuaternionDT=off  QuaternionDDT=off  QuaternionUnits=off  OutputVector=[1]  ActiveIO=on  Width=1  DialogClass=MechanicalSensorBlock  Primitive=R1  Force=off  ForceUnits=N  Torque=on  TorqueUnits=N*m  ReferenceFrame=Absolute (World)  ReactionSensedSide=Base  ReactionReferenceFrame=Absolute (World)  ReactionForce=off  ReactionForceUnits=N  ReactionMoment=off  ReactionMomentUnits=N*m
  Weld : mblibv1/Joints/Weld  DialogController=MECH.DynMechDlgSource  PhysicalDomain=mechanical  SubClassName=Unknown  LeftPortType=blob  RightPortType=blob  LConnTagsString=__newl0  RConnTagsString=__newr0  UpdateFromCAD=on  NumSAPorts=0  CutJoint=off  MarkAsCut=off  Primitives=weld  PrimitiveProps=W$WORLD$[0.57735,0.57735,0.57735]$weld  DialogClass=JointBlock  WAxis=[0.57735,0.57735,0.57735]
  Out_R1 : Outport
  Out_R2 : Outport  Port=2
  Out_R3 : Outport  Port=3
  Out_R4 : Outport  Port=4
  Out_R5 : Outport  Port=5
  Out_R6 : Outport  Port=6
  Out_End : Outport  Port=7
  wires:
  In_R1/1 -> Actuator1/1
  Sensor1/1 -> Out_R1/1
  In_R2/1 -> Actuator2/1
  Sensor2/1 -> Out_R2/1
  In_R3/1 -> Actuator3/1
  Sensor3/1 -> Out_R3/1
  Sensor4/1 -> Out_R4/1
  In_R4/1 -> Actuator4/1
  Sensor5/1 -> Out_R5/1
  In_R5/1 -> Actuator5/1
  Sensor6/1 -> Out_R6/1
  In_R6/1 -> Actuator6/1
  Body Sensor/1 -> Out_End/1
  connections:
  Body Sensor/LConn1 -- Body6/RConn1
  Sensor6/LConn1 -- R6/RConn2
  Actuator6/RConn1 -- R6/LConn3
  Weld/LConn1 -- Ground/RConn1
  Actuator3/RConn1 -- R3/LConn3
  Init3/RConn1 -- R3/LConn2
  Sensor3/LConn1 -- R3/RConn2
  Machine Environment/RConn1 -- Ground/LConn1
  R5/LConn1 -- Body4/RConn1
  R1/LConn1 -- Base/RConn1
  R6/RConn1 -- Body6/LConn1
  R5/RConn1 -- Body5/LConn1
  Body5/RConn1 -- R6/LConn1
  Body2/RConn1 -- R3/LConn1
  R2/RConn1 -- Body2/LConn1
  R2/LConn1 -- Body1/RConn1
  Weld/RConn1 -- Base/LConn1
  Actuator2/RConn1 -- R2/LConn3
  Init6/RConn1 -- R6/LConn2
  Body1/LConn1 -- R1/RConn1
  Sensor2/LConn1 -- R2/RConn2
  Init2/RConn1 -- R2/LConn2
  R1/RConn2 -- Sensor1/LConn1
  Actuator1/RConn1 -- R1/LConn3
  R1/LConn2 -- Init1/RConn1
  Sensor5/LConn1 -- R5/RConn2
  R3/RConn1 -- Body3/LConn1
  Actuator5/RConn1 -- R5/LConn3
  Init5/RConn1 -- R5/LConn2
  R4/RConn1 -- Body4/LConn1
  R4/LConn1 -- Body3/RConn1
  Actuator4/RConn1 -- R4/LConn3
  Initi4/RConn1 -- R4/LConn2
  Sensor4/LConn1 -- R4/RConn2

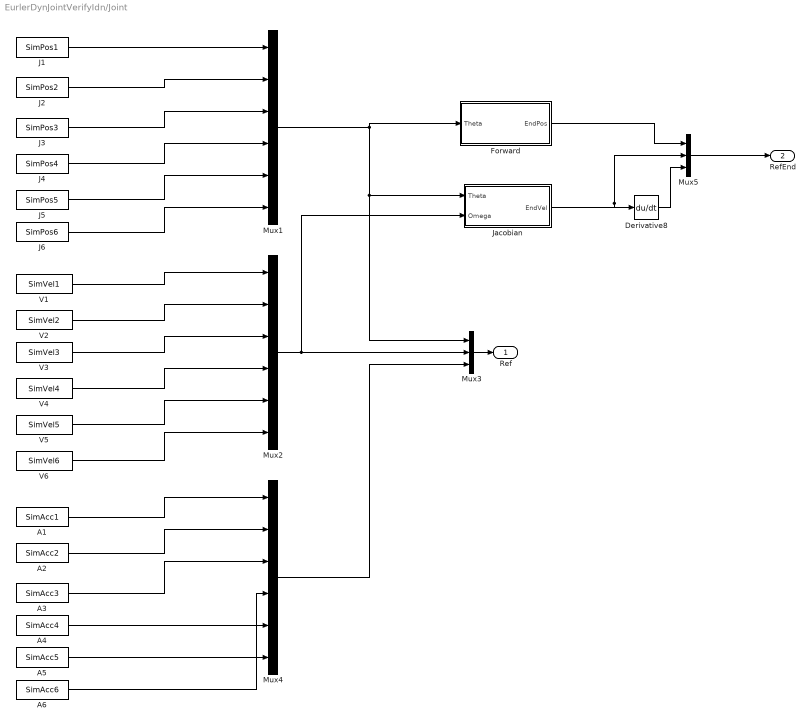
== system EurlerDynJointVerifyIdn/Joint ==
  A1 : FromWorkspace  VariableName=SimAcc1  SampleTime=4e-3
  A2 : FromWorkspace  VariableName=SimAcc2  SampleTime=4e-3
  A3 : FromWorkspace  VariableName=SimAcc3  SampleTime=4e-3
  A4 : FromWorkspace  VariableName=SimAcc4  SampleTime=4e-3
  A5 : FromWorkspace  VariableName=SimAcc5  SampleTime=4e-3
  A6 : FromWorkspace  VariableName=SimAcc6  SampleTime=4e-3
  Derivative8 : Derivative
  Forward : Stateflow chart  TreatAsAtomicUnit=on
  J1 : FromWorkspace  VariableName=SimPos1  SampleTime=4e-3
  J2 : FromWorkspace  VariableName=SimPos2  SampleTime=4e-3
  J3 : FromWorkspace  VariableName=SimPos3  SampleTime=4e-3
  J4 : FromWorkspace  VariableName=SimPos4  SampleTime=4e-3
  J5 : FromWorkspace  VariableName=SimPos5  SampleTime=4e-3
  J6 : FromWorkspace  VariableName=SimPos6  SampleTime=4e-3
  Jacobian : Stateflow chart  TreatAsAtomicUnit=on
  Mux1 : Mux  Inputs=6
  Mux2 : Mux  Inputs=6
  Mux3 : Mux  Inputs=3
  Mux4 : Mux  Inputs=6
  Mux5 : Mux  Inputs=3
  V1 : FromWorkspace  VariableName=SimVel1  SampleTime=4e-3
  V2 : FromWorkspace  VariableName=SimVel2  SampleTime=4e-3
  V3 : FromWorkspace  VariableName=SimVel3  SampleTime=4e-3
  V4 : FromWorkspace  VariableName=SimVel4  SampleTime=4e-3
  V5 : FromWorkspace  VariableName=SimVel5  SampleTime=4e-3
  V6 : FromWorkspace  VariableName=SimVel6  SampleTime=4e-3
  Ref : Outport
  RefEnd : Outport  Port=2
  wires:
  Jacobian/1(EndVel) -> Mux5/2, Derivative8/1
  Mux3/1 -> Ref/1
  Mux2/1 -> Mux3/2, Jacobian/2(Omega)
  Mux1/1 -> Forward/1(Theta), Mux3/1, Jacobian/1(Theta)
  Mux4/1 -> Mux3/3
  Mux5/1 -> RefEnd/1
  Forward/1(EndPos) -> Mux5/1
  J1/1 -> Mux1/1
  J2/1 -> Mux1/2
  J3/1 -> Mux1/3
  J4/1 -> Mux1/4
  J5/1 -> Mux1/5
  J6/1 -> Mux1/6
  V1/1 -> Mux2/1
  V2/1 -> Mux2/2
  V3/1 -> Mux2/3
  V4/1 -> Mux2/4
  V5/1 -> Mux2/5
  V6/1 -> Mux2/6
  A1/1 -> Mux4/1
  A2/1 -> Mux4/2
  A3/1 -> Mux4/3
  A4/1 -> Mux4/4
  A5/1 -> Mux4/5
  A6/1 -> Mux4/6
  Derivative8/1 -> Mux5/3

== system EurlerDynJointVerifyIdn/KinematicMotionControl ==
  In1 : Inport
  Demux1 : Demux  Outputs=3
  Demux2 : Demux  Outputs=6
  Demux3 : Demux  Outputs=6
  Demux4 : Demux  Outputs=6
  Mux{1..6} (6 alike) : Mux  Inputs=3
  Out1 : Outport
  Out2 : Outport  Port=2
  Out3 : Outport  Port=3
  Out4 : Outport  Port=4
  Out5 : Outport  Port=5
  Out6 : Outport  Port=6
  wires:
  Demux1/3 -> Demux4/1
  Demux1/2 -> Demux3/1
  Demux1/1 -> Demux2/1
  Mux1/1 -> Out1/1
  Mux4/1 -> Out2/1
  Mux2/1 -> Out3/1
  In1/1 -> Demux1/1
  Mux3/1 -> Out4/1
  Mux5/1 -> Out5/1
  Mux6/1 -> Out6/1
  Demux2/1 -> Mux1/1
  Demux2/2 -> Mux4/1
  Demux2/3 -> Mux2/1
  Demux2/4 -> Mux3/1
  Demux2/5 -> Mux5/1
  Demux2/6 -> Mux6/1
  Demux3/1 -> Mux1/2
  Demux3/2 -> Mux4/2
  Demux3/3 -> Mux2/2
  Demux3/4 -> Mux3/2
  Demux3/5 -> Mux5/2
  Demux3/6 -> Mux6/2
  Demux4/1 -> Mux1/3
  Demux4/2 -> Mux4/3
  Demux4/3 -> Mux2/3
  Demux4/4 -> Mux3/3
  Demux4/5 -> Mux5/3
  Demux4/6 -> Mux6/3

== system EurlerDynJointVerifyIdn/Line ==
  Derivative{,1..3} (4 alike) : Derivative
  EndVelocity : Subsystem
  Integrator : Integrator  InitialCondition=init_Endx
  Integrator1 : Integrator  InitialCondition=init_Endy
  Integrator2 : Integrator  InitialCondition=init_Endz
  Inverse Kinematic : Stateflow chart  TreatAsAtomicUnit=on
  Jacobian : Stateflow chart  TreatAsAtomicUnit=on
  Mux{1..6} (6 alike) : Mux  Inputs=3
  Ref : Outport
  RefEnd : Outport  Port=2
  wires:
  Derivative3/1 -> Mux6/3
  Derivative2/1 -> Mux6/2
  Derivative1/1 -> Mux6/1
  Mux6/1 -> Mux4/3
  Mux4/1 -> RefEnd/1
  Mux5/1 -> Mux4/2
  Inverse Kinematic/1(theta) -> Jacobian/2(Theta), Mux3/1
  Derivative/1 -> Mux3/3
  Mux3/1 -> Ref/1
  Jacobian/1(Omega) -> Derivative/1, Mux3/2
  Mux1/1 -> Jacobian/1(EndVel)
  Mux2/1 -> Inverse Kinematic/1(EndPos), Mux4/1
  Integrator2/1 -> Mux2/3
  EndVelocity/3(EndVz) -> Derivative3/1, Mux5/3, Mux1/3, Integrator2/1
  EndVelocity/2(EndVy) -> Derivative2/1, Mux5/2, Mux1/2, Integrator1/1
  EndVelocity/1(EndVx) -> Derivative1/1, Mux5/1, Mux1/1, Integrator/1
  Integrator1/1 -> Mux2/2
  Integrator/1 -> Mux2/1

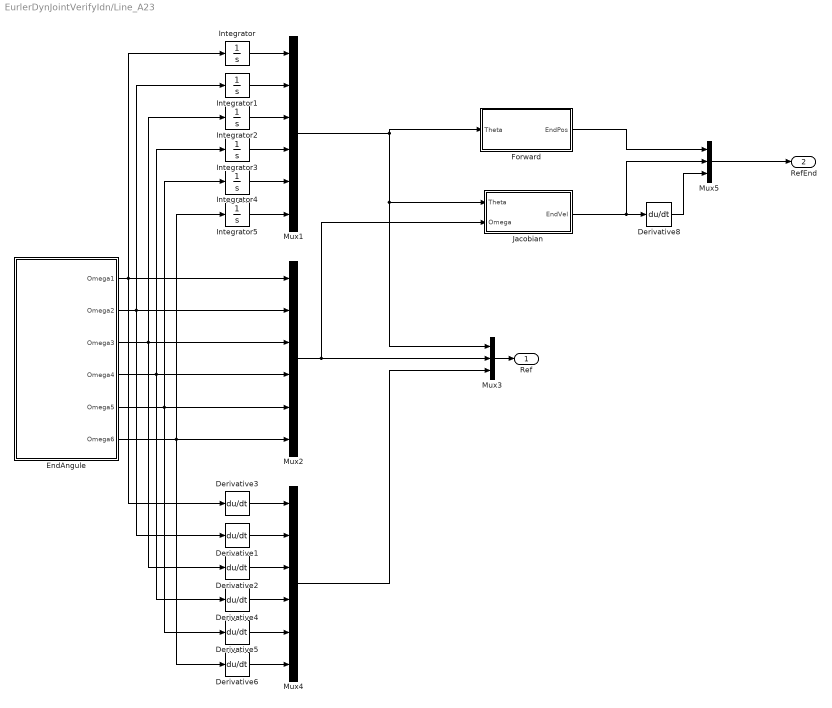
== system EurlerDynJointVerifyIdn/Line_A23 ==
  Derivative{1..6,8} (7 alike) : Derivative
  EndAngule : Subsystem
  Forward : Stateflow chart  TreatAsAtomicUnit=on
  Integrator : Integrator  InitialCondition=a1/180*pi
  Integrator1 : Integrator  InitialCondition=a2/180*pi
  Integrator2 : Integrator  InitialCondition=a3/180*pi
  Integrator3 : Integrator  InitialCondition=a4/180*pi
  Integrator4 : Integrator  InitialCondition=a5/180*pi
  Integrator5 : Integrator  InitialCondition=a6/180*pi
  Jacobian : Stateflow chart  TreatAsAtomicUnit=on
  Mux1 : Mux  Inputs=6
  Mux2 : Mux  Inputs=6
  Mux3 : Mux  Inputs=3
  Mux4 : Mux  Inputs=6
  Mux5 : Mux  Inputs=3
  Ref : Outport
  RefEnd : Outport  Port=2
  wires:
  Mux3/1 -> Ref/1
  EndAngule/1(Omega1) -> Integrator/1, Mux2/1, Derivative3/1
  EndAngule/2(Omega2) -> Integrator1/1, Mux2/2, Derivative1/1
  EndAngule/3(Omega3) -> Integrator2/1, Mux2/3, Derivative2/1
  EndAngule/4(Omega4) -> Integrator3/1, Mux2/4, Derivative4/1
  EndAngule/5(Omega5) -> Integrator4/1, Mux2/5, Derivative5/1
  EndAngule/6(Omega6) -> Integrator5/1, Mux2/6, Derivative6/1
  Integrator/1 -> Mux1/1
  Integrator1/1 -> Mux1/2
  Integrator2/1 -> Mux1/3
  Integrator3/1 -> Mux1/4
  Integrator4/1 -> Mux1/5
  Integrator5/1 -> Mux1/6
  Derivative3/1 -> Mux4/1
  Derivative1/1 -> Mux4/2
  Derivative2/1 -> Mux4/3
  Derivative4/1 -> Mux4/4
  Derivative5/1 -> Mux4/5
  Derivative6/1 -> Mux4/6
  Mux2/1 -> Mux3/2, Jacobian/2(Omega)
  Mux1/1 -> Forward/1(Theta), Mux3/1, Jacobian/1(Theta)
  Mux4/1 -> Mux3/3
  Mux5/1 -> RefEnd/1
  Forward/1(EndPos) -> Mux5/1
  Jacobian/1(EndVel) -> Mux5/2, Derivative8/1
  Derivative8/1 -> Mux5/3

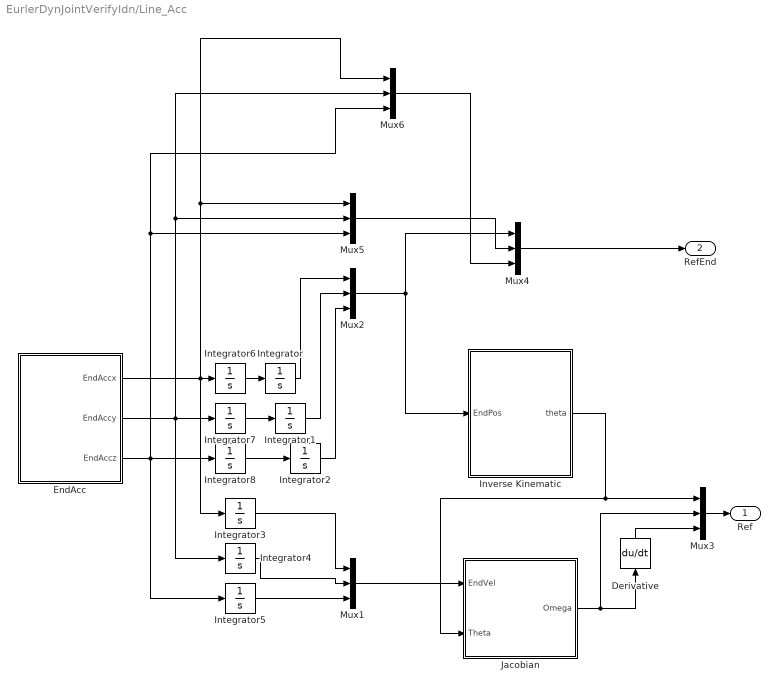
== system EurlerDynJointVerifyIdn/Line_Acc ==
  Derivative : Derivative
  EndAcc : Subsystem
  Integrator : Integrator  InitialCondition=init_Endx
  Integrator1 : Integrator  InitialCondition=init_Endy
  Integrator2 : Integrator  InitialCondition=init_Endz
  Integrator{3..4,6..7} (4 alike) : Integrator  InitialCondition=30
  Integrator5 : Integrator  InitialCondition=-30
  Integrator8 : Integrator  InitialCondition=-30
  Inverse Kinematic : Stateflow chart  TreatAsAtomicUnit=on
  Jacobian : Stateflow chart  TreatAsAtomicUnit=on
  Mux{1..6} (6 alike) : Mux  Inputs=3
  Ref : Outport
  RefEnd : Outport  Port=2
  wires:
  Integrator/1 -> Mux2/1
  Integrator1/1 -> Mux2/2
  EndAcc/1(EndAccx) -> Mux5/1, Mux6/1, Integrator3/1, Integrator6/1
  EndAcc/2(EndAccy) -> Mux5/2, Mux6/2, Integrator4/1, Integrator7/1
  EndAcc/3(EndAccz) -> Mux5/3, Mux6/3, Integrator5/1, Integrator8/1
  Integrator2/1 -> Mux2/3
  Mux2/1 -> Mux4/1, Inverse Kinematic/1(EndPos)
  Mux1/1 -> Jacobian/1(EndVel)
  Jacobian/1(Omega) -> Mux3/2, Derivative/1
  Mux3/1 -> Ref/1
  Derivative/1 -> Mux3/3
  Inverse Kinematic/1(theta) -> Mux3/1, Jacobian/2(Theta)
  Mux5/1 -> Mux4/2
  Mux4/1 -> RefEnd/1
  Mux6/1 -> Mux4/3
  Integrator3/1 -> Mux1/1
  Integrator4/1 -> Mux1/2
  Integrator5/1 -> Mux1/3
  Integrator6/1 -> Integrator/1
  Integrator7/1 -> Integrator1/1
  Integrator8/1 -> Integrator2/1

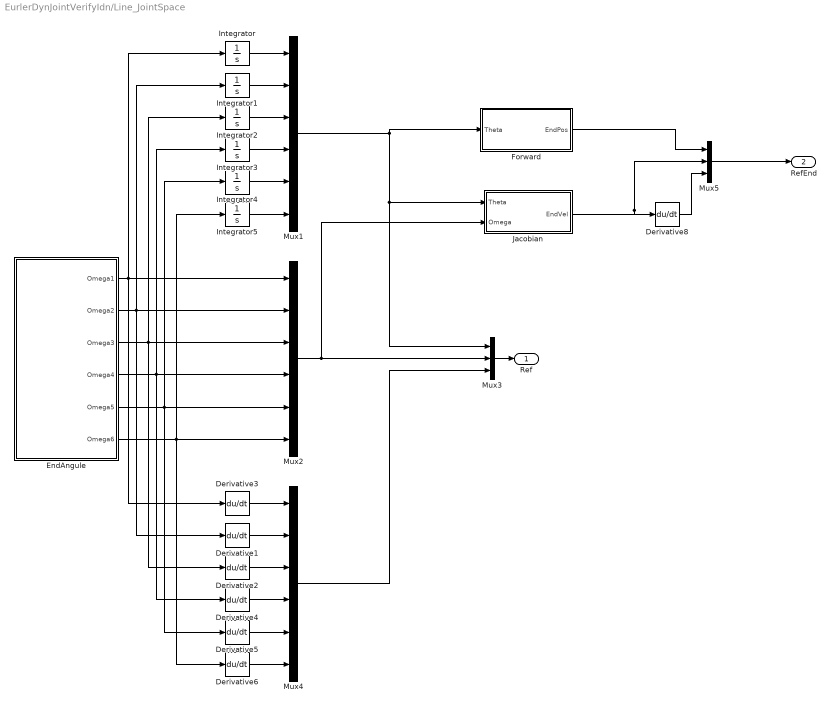
== system EurlerDynJointVerifyIdn/Line_JointSpace ==
  Derivative{1..6,8} (7 alike) : Derivative
  EndAngule : Subsystem
  Forward : Stateflow chart  TreatAsAtomicUnit=on
  Integrator : Integrator  InitialCondition=a1/180*pi
  Integrator1 : Integrator  InitialCondition=a2/180*pi
  Integrator2 : Integrator  InitialCondition=a3/180*pi
  Integrator3 : Integrator  InitialCondition=a4/180*pi
  Integrator4 : Integrator  InitialCondition=a5/180*pi
  Integrator5 : Integrator  InitialCondition=a6/180*pi
  Jacobian : Stateflow chart  TreatAsAtomicUnit=on
  Mux1 : Mux  Inputs=6
  Mux2 : Mux  Inputs=6
  Mux3 : Mux  Inputs=3
  Mux4 : Mux  Inputs=6
  Mux5 : Mux  Inputs=3
  Ref : Outport
  RefEnd : Outport  Port=2
  wires:
  Derivative8/1 -> Mux5/3
  Forward/1(EndPos) -> Mux5/1
  Mux5/1 -> RefEnd/1
  Mux4/1 -> Mux3/3
  Mux1/1 -> Jacobian/1(Theta), Mux3/1, Forward/1(Theta)
  Mux2/1 -> Jacobian/2(Omega), Mux3/2
  Derivative6/1 -> Mux4/6
  Derivative5/1 -> Mux4/5
  Derivative4/1 -> Mux4/4
  Derivative2/1 -> Mux4/3
  Derivative1/1 -> Mux4/2
  Derivative3/1 -> Mux4/1
  Integrator5/1 -> Mux1/6
  Integrator4/1 -> Mux1/5
  Integrator3/1 -> Mux1/4
  Integrator2/1 -> Mux1/3
  Integrator1/1 -> Mux1/2
  Integrator/1 -> Mux1/1
  EndAngule/6(Omega6) -> Derivative6/1, Mux2/6, Integrator5/1
  EndAngule/5(Omega5) -> Derivative5/1, Mux2/5, Integrator4/1
  EndAngule/4(Omega4) -> Derivative4/1, Mux2/4, Integrator3/1
  EndAngule/3(Omega3) -> Derivative2/1, Mux2/3, Integrator2/1
  EndAngule/2(Omega2) -> Derivative1/1, Mux2/2, Integrator1/1
  EndAngule/1(Omega1) -> Derivative3/1, Mux2/1, Integrator/1
  Mux3/1 -> Ref/1
  Jacobian/1(EndVel) -> Mux5/2, Derivative8/1

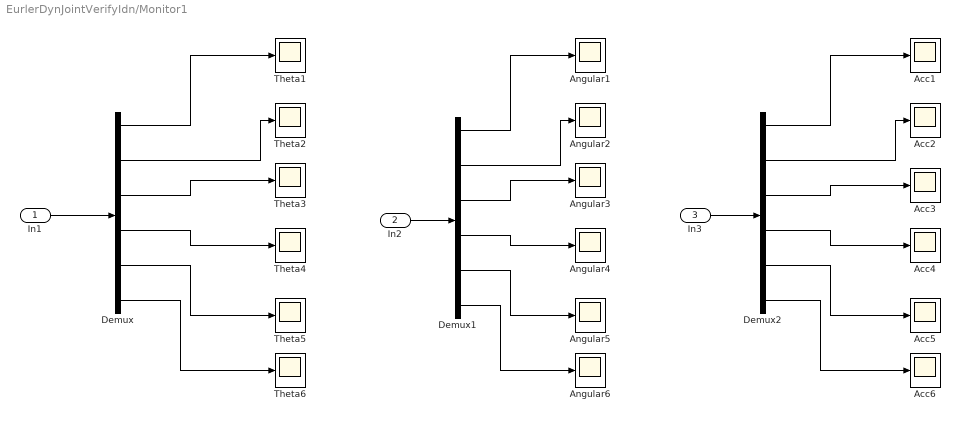
== system EurlerDynJointVerifyIdn/Monitor1 ==
  In1 : Inport
  In2 : Inport  Port=2
  In3 : Inport  Port=3
  Acc{1..6} (6 alike) : Scope
      Acc1 settings: TimeRange=10  SaveName=ScopeData33
      Acc2 settings: SaveName=ScopeData34
      Acc3 settings: SaveName=ScopeData35
      Acc4 settings: SaveName=ScopeData36
      Acc5 settings: SaveName=ScopeData37
      Acc6 settings: SaveName=ScopeData38
  Angular{1..6} (6 alike) : Scope
      Angular1 settings: SaveName=ScopeData27
      Angular2 settings: SaveName=ScopeData28
      Angular3 settings: SaveName=ScopeData29
      Angular4 settings: SaveName=ScopeData30
      Angular5 settings: SaveName=ScopeData31
      Angular6 settings: SaveName=ScopeData32
  Demux : Demux  Outputs=6
  Demux1 : Demux  Outputs=6
  Demux2 : Demux  Outputs=6
  Theta{1..6} (6 alike) : Scope
      Theta1 settings: SaveName=ScopeData22
      Theta2 settings: SaveName=ScopeData21
      Theta3 settings: SaveName=ScopeData23
      Theta4 settings: SaveName=ScopeData24
      Theta5 settings: SaveName=ScopeData25
      Theta6 settings: SaveName=ScopeData26
  wires:
  In1/1 -> Demux/1
  In2/1 -> Demux1/1
  In3/1 -> Demux2/1
  Demux/1 -> Theta1/1
  Demux/2 -> Theta2/1
  Demux/3 -> Theta3/1
  Demux/4 -> Theta4/1
  Demux/5 -> Theta5/1
  Demux/6 -> Theta6/1
  Demux1/1 -> Angular1/1
  Demux1/2 -> Angular2/1
  Demux1/3 -> Angular3/1
  Demux1/4 -> Angular4/1
  Demux1/5 -> Angular5/1
  Demux1/6 -> Angular6/1
  Demux2/1 -> Acc1/1
  Demux2/2 -> Acc2/1
  Demux2/3 -> Acc3/1
  Demux2/4 -> Acc4/1
  Demux2/5 -> Acc5/1
  Demux2/6 -> Acc6/1

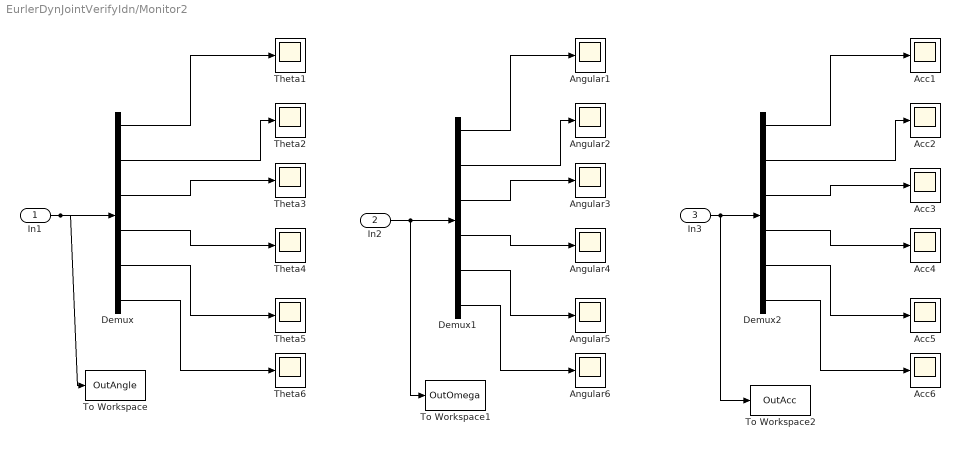
== system EurlerDynJointVerifyIdn/Monitor2 ==
  In1 : Inport
  In2 : Inport  Port=2
  In3 : Inport  Port=3
  Acc{1..6} (6 alike) : Scope
      Acc1 settings: TimeRange=10  SaveName=ScopeData33
      Acc2 settings: SaveName=ScopeData34
      Acc3 settings: SaveName=ScopeData35
      Acc4 settings: SaveName=ScopeData36
      Acc5 settings: SaveName=ScopeData37
      Acc6 settings: SaveName=ScopeData38
  Angular{1..6} (6 alike) : Scope
      Angular1 settings: SaveName=ScopeData27
      Angular2 settings: SaveName=ScopeData28
      Angular3 settings: SaveName=ScopeData29
      Angular4 settings: SaveName=ScopeData30
      Angular5 settings: SaveName=ScopeData31
      Angular6 settings: SaveName=ScopeData32
  Demux : Demux  Outputs=6
  Demux1 : Demux  Outputs=6
  Demux2 : Demux  Outputs=6
  Theta{1..6} (6 alike) : Scope
      Theta1 settings: SaveName=ScopeData22
      Theta2 settings: SaveName=ScopeData21
      Theta3 settings: SaveName=ScopeData23
      Theta4 settings: SaveName=ScopeData24
      Theta5 settings: SaveName=ScopeData25
      Theta6 settings: SaveName=ScopeData26
  To Workspace : ToWorkspace  VariableName=OutAngle  SampleTime=-1  SaveFormat=Structure
  To Workspace1 : ToWorkspace  VariableName=OutOmega  SampleTime=-1  SaveFormat=Structure
  To Workspace2 : ToWorkspace  VariableName=OutAcc  SampleTime=-1  SaveFormat=Structure
  wires:
  In1/1 -> Demux/1, To Workspace/1
  In2/1 -> Demux1/1, To Workspace1/1
  In3/1 -> Demux2/1, To Workspace2/1
  Demux/1 -> Theta1/1
  Demux/2 -> Theta2/1
  Demux/3 -> Theta3/1
  Demux/4 -> Theta4/1
  Demux/5 -> Theta5/1
  Demux/6 -> Theta6/1
  Demux1/1 -> Angular1/1
  Demux1/2 -> Angular2/1
  Demux1/3 -> Angular3/1
  Demux1/4 -> Angular4/1
  Demux1/5 -> Angular5/1
  Demux1/6 -> Angular6/1
  Demux2/1 -> Acc1/1
  Demux2/2 -> Acc2/1
  Demux2/3 -> Acc3/1
  Demux2/4 -> Acc4/1
  Demux2/5 -> Acc5/1
  Demux2/6 -> Acc6/1

== system EurlerDynJointVerifyIdn/Still ==
  Derivative : Derivative
  Derivative1 : Derivative
  Derivative3 : Derivative
  Drivative2 : Derivative
  EndVelocity : Subsystem
  Integrator : Integrator  InitialCondition=init_Endx
  Integrator1 : Integrator  InitialCondition=init_Endy
  Integrator2 : Integrator  InitialCondition=init_Endz
  Inverse Kinematic : Stateflow chart  TreatAsAtomicUnit=on
  Jacobian : Stateflow chart  TreatAsAtomicUnit=on
  Mux{1..6} (6 alike) : Mux  Inputs=3
  Ref : Outport
  RefEnd : Outport  Port=2
  wires:
  Integrator/1 -> Mux2/1
  Integrator1/1 -> Mux2/2
  EndVelocity/1(EndVx) -> Integrator/1, Mux1/1, Mux5/1, Derivative1/1
  EndVelocity/2(EndVy) -> Integrator1/1, Mux1/2, Mux5/2, Drivative2/1
  EndVelocity/3(EndVz) -> Integrator2/1, Mux1/3, Mux5/3, Derivative3/1
  Integrator2/1 -> Mux2/3
  Mux2/1 -> Mux4/1, Inverse Kinematic/1(EndPos)
  Mux1/1 -> Jacobian/1(EndVel)
  Jacobian/1(Omega) -> Mux3/2, Derivative/1
  Mux3/1 -> Ref/1
  Derivative/1 -> Mux3/3
  Inverse Kinematic/1(theta) -> Mux3/1, Jacobian/2(Theta)
  Mux5/1 -> Mux4/2
  Mux4/1 -> RefEnd/1
  Derivative1/1 -> Mux6/1
  Drivative2/1 -> Mux6/2
  Derivative3/1 -> Mux6/3
  Mux6/1 -> Mux4/3

== system EurlerDynJointVerifyIdn/Circle_XY/EndVelocity ==
  Constant : Constant  Value=-1
  End_Vx : Sin  Amplitude=-tvel  Frequency=freq  SampleTime=0
  End_Vy : Sin  Frequency=freq  Phase=pi/2  SampleTime=0
  End_Vz : Constant  Value=0
  Gain : Gain  Gain=tvel
  Ramp : simulink/Sources/Ramp  SystemSampleTime=-1  slope=1  start=0  X0=0
  Ramp1 : simulink/Sources/Ramp  SystemSampleTime=-1  slope=-1  start=1  X0=0
  Sum : Sum  Inputs=|++
  Sum1 : Sum  Inputs=++|
  Sum2 : Sum  Inputs=++|
  Transport Delay : TransportDelay
  Transport Delay1 : TransportDelay
  EndVx : Outport
  EndVy : Outport  Port=2
  EndVz : Outport  Port=3
  wires:
  End_Vy/1 -> Sum2/1
  Ramp/1 -> Sum/1
  Ramp1/1 -> Sum/2
  Transport Delay/1 -> Sum1/1
  Sum2/1 -> Transport Delay/1
  Constant/1 -> Sum2/2
  Sum/1 -> Sum1/2
  Sum1/1 -> Gain/1
  End_Vx/1 -> Transport Delay1/1
  Gain/1 -> EndVy/1
  End_Vz/1 -> EndVx/1
  Transport Delay1/1 -> EndVz/1

== system EurlerDynJointVerifyIdn/Circle_XZ/EndVelocity ==
  Constant : Constant  Value=-1
  End_Vx : Sin  Amplitude=-tvel  Frequency=freq  SampleTime=0
  End_Vy : Sin  Frequency=freq  Phase=pi/2  SampleTime=0
  End_Vz : Constant  Value=0
  Gain : Gain  Gain=tvel
  Ramp : simulink/Sources/Ramp  SystemSampleTime=-1  slope=1  start=0  X0=0
  Ramp1 : simulink/Sources/Ramp  SystemSampleTime=-1  slope=-1  start=1  X0=0
  Sum : Sum  Inputs=|++
  Sum1 : Sum  Inputs=++|
  Sum2 : Sum  Inputs=++|
  Transport Delay : TransportDelay
  Transport Delay1 : TransportDelay
  EndVx : Outport
  EndVy : Outport  Port=2
  EndVz : Outport  Port=3
  wires:
  End_Vy/1 -> Sum2/1
  Ramp/1 -> Sum/1
  Ramp1/1 -> Sum/2
  Transport Delay/1 -> Sum1/1
  Sum2/1 -> Transport Delay/1
  Constant/1 -> Sum2/2
  Sum/1 -> Sum1/2
  Sum1/1 -> Gain/1
  End_Vx/1 -> Transport Delay1/1
  Transport Delay1/1 -> EndVx/1
  Gain/1 -> EndVz/1
  End_Vz/1 -> EndVy/1
